simulink model "sampleModel1761"  (R2023a)
settings: Solver=VariableStepAuto  StartTime=0.0  StopTime=10.0  RelTol=1e-3
libraries: hdlsllib x3, simulink x1
settings Model: Creator=user1  LastModifiedBy=user1

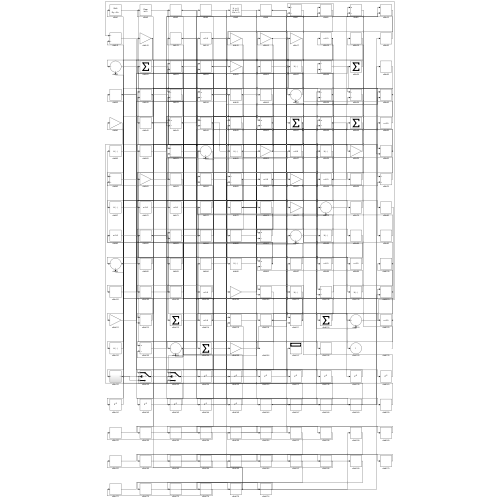
[thumbnail: Simulink's stored preview of the top-level diagram]
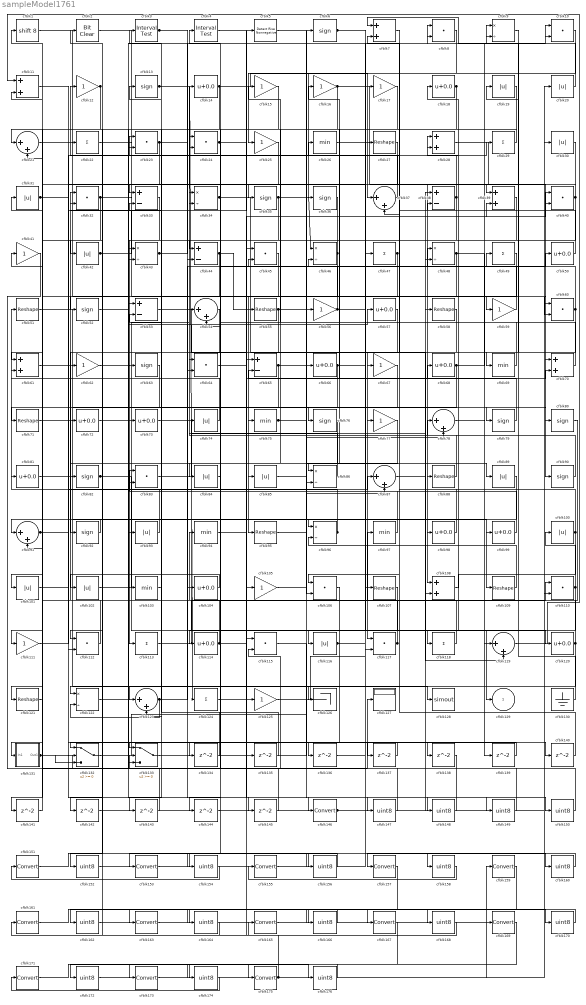
== system sampleModel1761 ==
  cfblk1 : ArithShift  BitShiftNumber=8
  cfblk{8,10,23..24,32,40,45,60,64,83,106,110,112,115,117} (15 alike) : DotProduct  OutDataTypeStr=Inherit: Inherit via internal rule
  cfblk{19..20,30..31,42,74,84..85,89,93,100..102,116} (14 alike) : Abs  SaturateOnIntegerOverflow=off
  cfblk{26,69,75,94,97,103} (6 alike) : MinMax
  cfblk{14,18,50,57,66,68,72..73,81,98..99,104,114,120} (14 alike) : Bias  Bias=0.0  SaturateOnIntegerOverflow=off
  cfblk{12,15..17,25,41,56,59,62,67,77,105,111,125} (14 alike) : Gain
  cfblk{27,51,55,58,71,88,95,107,109,121} (10 alike) : Reshape
  cfblk{7,11,28,39,61,70,108} (7 alike) : Sum
  cfblk{22,29,47,49,113,118,124} (7 alike) : Sum  Inputs=+
  cfblk{21,37,54,78,87,91,119,123} (8 alike) : Sum  Inputs=|++
  cfblk{9,34,43,46,48,86,96,122} (8 alike) : Product  Inputs=*/  RndMeth=Zero  SaturateOnIntegerOverflow=on
  cfblk126 : Terminator
  cfblk127 : Display
  cfblk128 : ToWorkspace  VariableName=simout  SaveFormat=Timeseries  SampleTime=-1
  cfblk{6,13,35..36,52,63,76,79..80,82,90,92} (12 alike) : Signum
  cfblk130 : Ground
  cfblk131 : Subsystem
      settings: LibrarySourceBlock=|
      | hdlsllib/Ports &
      | Subsystems/Subsystem
  cfblk132 : Switch  SaturateOnIntegerOverflow=off  InputSameDT=off
  cfblk133 : Switch  SaturateOnIntegerOverflow=off  InputSameDT=off
  cfblk{134..145} (12 alike) : Delay  SampleTime=1
  cfblk{146,151,153,155,157,159,161,163,165,167,169,171,173,175} (14 alike) : DataTypeConversion  SaturateOnIntegerOverflow=off  RndMeth=Floor
  cfblk{147..150,152,154,156,158,160,162,164,166,168,170,172,174,176} (17 alike) : DataTypeConversion  OutDataTypeStr=uint8  SaturateOnIntegerOverflow=off  RndMeth=Floor
  cfblk2 : simulink/Logic and Bit Operations/Bit Clear  iBit=0
      settings: LibrarySourceBlock=|
      | hdlsllib/Logic and Bit
      | Operations/Bit Clear
  cfblk3 : hdlsllib/Logic and Bit Operations/Interval Test  IntervalClosedRight=on  uplimit=0.5  IntervalClosedLeft=on  lowlimit=-0.5  OutDataTypeStr=boolean
  cfblk{33,38,44,53,65} (5 alike) : Sum  Inputs=+-
  cfblk4 : hdlsllib/Logic and Bit Operations/Interval Test  IntervalClosedRight=on  uplimit=0.5  IntervalClosedLeft=on  lowlimit=-0.5  OutDataTypeStr=boolean
  cfblk5 : hdlsllib/Logic and Bit Operations/Detect Rise Nonnegative  vinit=0  OutDataTypeStr=boolean
  cfblk129 : Outport  VectorParamsAs1DForOutWhenUnconnected=off
  wires:
  cfblk61/1 -> cfblk128/1
  cfblk39/1 -> cfblk113/1
  cfblk1/1 -> cfblk53/1
  cfblk13/1 -> cfblk124/1, cfblk138/1
  cfblk93/1 -> cfblk51/1
  cfblk81/1 -> cfblk96/1
  cfblk76/1 -> cfblk123/1
  cfblk133/1 -> cfblk66/1
  cfblk117/1 -> cfblk32/1, cfblk81/1
  cfblk41/1 -> cfblk127/1
  cfblk42/1 -> cfblk95/1, cfblk5/1
  cfblk15/1 -> cfblk112/1
  cfblk14/1 -> cfblk37/1, cfblk72/1, cfblk80/1
  cfblk22/1 -> cfblk108/1
  cfblk132/1 -> cfblk56/1
  cfblk16/1 -> cfblk98/1, cfblk43/2
  cfblk28/1 -> cfblk90/1
  cfblk29/1 -> cfblk21/1
  cfblk12/1 -> cfblk131/1(In1), cfblk132/2
  cfblk92/1 -> cfblk91/1
  cfblk88/1 -> cfblk14/1
  cfblk85/1 -> cfblk6/1
  cfblk8/1 -> cfblk25/1
  cfblk123/1 -> cfblk49/1, cfblk122/2
  cfblk51/1 -> cfblk79/1
  cfblk20/1 -> cfblk7/1
  cfblk102/1 -> cfblk34/1
  cfblk73/1 -> cfblk116/1
  cfblk32/1 -> cfblk88/1, cfblk111/1
  cfblk86/1 -> cfblk74/1
  cfblk77/1 -> cfblk92/1
  cfblk108/1 -> cfblk28/1
  cfblk47/1 -> cfblk61/1, cfblk75/1
  cfblk67/1 -> cfblk101/1
  cfblk63/1 -> cfblk121/1
  cfblk21/1 -> cfblk47/1
  cfblk27/1 -> cfblk42/1
  cfblk66/1 -> cfblk123/2, cfblk40/2
  cfblk26/1 -> cfblk70/1
  cfblk80/1 -> cfblk106/1
  cfblk118/1 -> cfblk94/1
  cfblk2/1 -> cfblk104/1
  cfblk69/1 -> cfblk15/1
  cfblk43/1 -> cfblk73/1, cfblk8/1
  cfblk44/1 -> cfblk55/1, cfblk142/1
  cfblk104/1 -> cfblk102/1
  cfblk52/1 -> cfblk9/1
  cfblk34/1 -> cfblk117/1, cfblk108/2
  cfblk7/1 -> cfblk67/1
  cfblk109/1 -> cfblk96/2
  cfblk113/1 -> cfblk97/1
  cfblk91/1 -> cfblk34/2, cfblk21/2
  cfblk99/1 -> cfblk83/1
  cfblk46/1 -> cfblk44/1, cfblk143/1
  cfblk97/1 -> cfblk13/1
  cfblk119/1 -> cfblk11/1
  cfblk122/1 -> cfblk57/1
  cfblk19/1 -> cfblk76/1
  cfblk95/1 -> cfblk68/1
  cfblk82/1 -> cfblk129/1, cfblk8/2
  cfblk35/1 -> cfblk46/1, cfblk144/1
  cfblk120/1 -> cfblk3/1, cfblk152/1
  cfblk25/1 -> cfblk52/1
  cfblk116/1 -> cfblk10/1, cfblk110/1
  cfblk74/1 -> cfblk41/1
  cfblk40/1 -> cfblk33/1, cfblk63/1
  cfblk71/1 -> cfblk109/1
  cfblk10/1 -> cfblk36/1
  cfblk110/1 -> cfblk100/1, cfblk126/1
  cfblk89/1 -> cfblk112/2
  cfblk96/1 -> cfblk11/2, cfblk24/2
  cfblk23/1 -> cfblk71/1, cfblk150/1
  cfblk4/1 -> cfblk146/1
  cfblk125/1 -> cfblk27/1
  cfblk121/1 -> cfblk61/2
  cfblk57/1 -> cfblk106/2
  cfblk84/1 -> cfblk64/1
  cfblk56/1 -> cfblk60/1, cfblk45/2, cfblk16/1
  cfblk130/1 -> cfblk9/2
  cfblk60/1 -> cfblk19/1, cfblk24/1, cfblk86/1
  cfblk37/1 -> cfblk12/1
  cfblk58/1 -> cfblk82/1
  cfblk31/1 -> cfblk35/1, cfblk147/1
  cfblk111/1 -> cfblk29/1
  cfblk53/1 -> cfblk125/1
  cfblk55/1 -> cfblk114/1, cfblk87/2
  cfblk90/1 -> cfblk78/1
  cfblk83/1 -> cfblk58/1
  cfblk9/1 -> cfblk39/1
  cfblk65/1 -> cfblk84/1, cfblk89/1, cfblk141/1
  cfblk75/1 -> cfblk50/1, cfblk99/1, cfblk78/2, cfblk48/1
  cfblk49/1 -> cfblk62/1
  cfblk5/1 -> cfblk60/2
  cfblk100/1 -> cfblk65/2, cfblk118/1
  cfblk24/1 -> cfblk105/1, cfblk59/1
  cfblk105/1 -> cfblk40/1
  cfblk54/1 -> cfblk64/2
  cfblk62/1 -> cfblk54/1
  cfblk36/1 -> cfblk54/2
  cfblk48/1 -> cfblk119/1, cfblk86/2
  cfblk101/1 -> cfblk87/1
  cfblk33/1 -> cfblk83/2
  cfblk50/1 -> cfblk23/1
  cfblk3/1 -> cfblk77/1, cfblk149/1
  cfblk112/1 -> cfblk31/1
  cfblk87/1 -> cfblk119/2
  cfblk94/1 -> cfblk70/2
  cfblk103/1 -> cfblk23/2
  cfblk98/1 -> cfblk7/2
  cfblk131/1(Out1) -> cfblk133/2, cfblk132/3
  cfblk70/1 -> cfblk22/1
  cfblk30/1 -> cfblk69/1
  cfblk6/1 -> cfblk107/1, cfblk120/1
  cfblk38/1 -> cfblk44/2, cfblk28/2
  cfblk114/1 -> cfblk33/2, cfblk39/2
  cfblk68/1 -> cfblk18/1, cfblk10/2, cfblk38/2, cfblk93/1
  cfblk59/1 -> cfblk26/1
  cfblk45/1 -> cfblk122/1
  cfblk79/1 -> cfblk46/2
  cfblk18/1 -> cfblk85/1, cfblk103/1
  cfblk107/1 -> cfblk134/1
  cfblk134/1 -> cfblk53/2
  cfblk64/1 -> cfblk135/1
  cfblk135/1 -> cfblk32/2
  cfblk106/1 -> cfblk136/1
  cfblk136/1 -> cfblk117/2
  cfblk124/1 -> cfblk137/1
  cfblk137/1 -> cfblk133/1
  cfblk138/1 -> cfblk133/3
  cfblk78/1 -> cfblk139/1
  cfblk139/1 -> cfblk132/1
  cfblk11/1 -> cfblk140/1
  cfblk140/1 -> cfblk37/2
  cfblk141/1 -> cfblk91/2
  cfblk142/1 -> cfblk65/1
  cfblk143/1 -> cfblk43/1
  cfblk144/1 -> cfblk110/2
  cfblk72/1 -> cfblk145/1
  cfblk145/1 -> cfblk1/1
  cfblk146/1 -> cfblk48/2, cfblk20/1
  cfblk147/1 -> cfblk4/1
  cfblk115/1 -> cfblk148/1
  cfblk148/1 -> cfblk38/1
  cfblk149/1 -> cfblk115/1
  cfblk150/1 -> cfblk115/2
  cfblk152/1 -> cfblk17/1
  cfblk17/1 -> cfblk154/1
  cfblk154/1 -> cfblk151/1
  cfblk151/1 -> cfblk156/1
  cfblk156/1 -> cfblk153/1
  cfblk153/1 -> cfblk158/1
  cfblk158/1 -> cfblk155/1
  cfblk155/1 -> cfblk160/1
  cfblk160/1 -> cfblk157/1
  cfblk157/1 -> cfblk162/1
  cfblk162/1 -> cfblk159/1
  cfblk159/1 -> cfblk164/1
  cfblk164/1 -> cfblk161/1
  cfblk161/1 -> cfblk166/1
  cfblk166/1 -> cfblk163/1
  cfblk163/1 -> cfblk168/1
  cfblk168/1 -> cfblk165/1
  cfblk165/1 -> cfblk170/1
  cfblk170/1 -> cfblk167/1
  cfblk167/1 -> cfblk172/1
  cfblk172/1 -> cfblk169/1
  cfblk173/1 -> cfblk175/1
  cfblk169/1 -> cfblk174/1
  cfblk174/1 -> cfblk171/1
  cfblk175/1 -> cfblk2/1, cfblk45/1, cfblk30/1
  cfblk171/1 -> cfblk176/1
  cfblk176/1 -> cfblk173/1

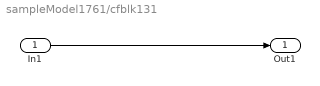
== system sampleModel1761/cfblk131 ==
  In1 : Inport
  Out1 : Outport
  wires:
  In1/1 -> Out1/1
